simulink model "PlantaMalhaExternaR2018b"  (R2018b)
settings: Solver=VariableStepAuto  StartTime=0.0  StopTime=10.0  RelTol=1e-3
libraries: simulink x1
settings Model: Creator=lucas  LastModifiedBy=vitor
settings DataIOCC: ReturnWorkspaceOutputs=on
settings DebuggingCC: SFMachineParentedDataDiag=error

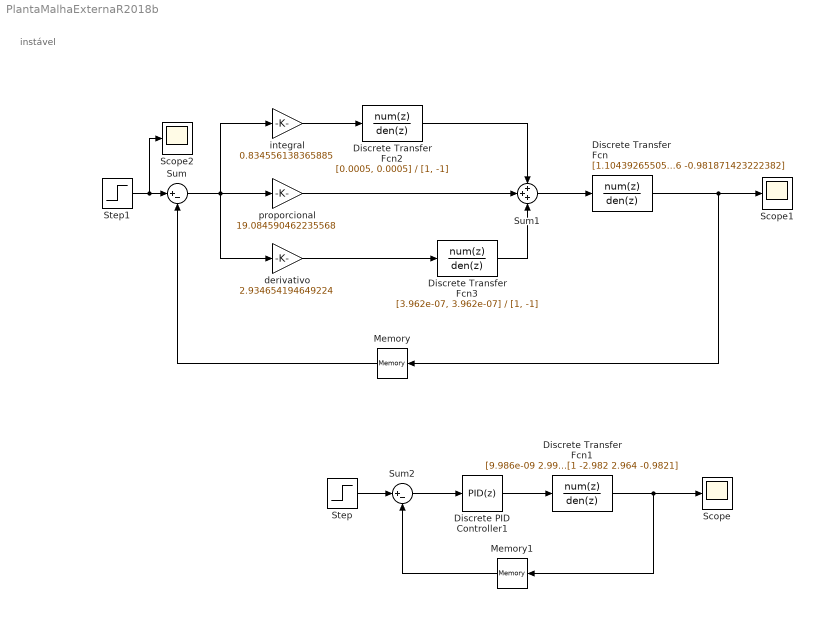
== system PlantaMalhaExternaR2018b ==
  note: instável
  Discrete Transfer Fcn : DiscreteTransferFcn  Numerator=[1.104392655054829e-08 3.313177965164485e-08 3.313177965164485e-08 1.104392655054829e-08]  Denominator=[1 -2.981694681338594 2.963566104560976 -0.981871423222382]  SampleTime=0.001
  Discrete Transfer Fcn1 : DiscreteTransferFcn  Numerator=[9.986e-09 2.996e-08 2.996e-08 9.986e-09]  Denominator=[1 -2.982 2.964 -0.9821]  SampleTime=0.001
  Discrete Transfer Fcn2 : DiscreteTransferFcn  Numerator=[0.0005, 0.0005]  Denominator=[1, -1]
  Discrete Transfer Fcn3 : DiscreteTransferFcn  Numerator=[3.962e-07, 3.962e-07]  Denominator=[1, -1]  SampleTime=0.001
  Discrete PID Controller1 : simulink/Continuous/PID Controller  Controller=PID  Form=Parallel  TimeDomain=Discrete-time  SampleTime=0.001  IntegratorMethod=Forward Euler  FilterMethod=Forward Euler  ControllerParametersSource=internal  P=200  I=0  D=8  UseFilter=on  N=1.824  TunerSelectOption=Transfer Function Based (PID Tuner App)  InitialConditionSource=internal  InitialConditionForIntegrator=0  InitialConditionForFilter=0  DifferentiatorICPrevScaledInput=0  ExternalReset=none  TrackingMode=off  Kt=1  LimitOutput=off  UpperSaturationLimit=inf  LowerSaturationLimit=-inf  LinearizeAsGain=off  AntiWindupMode=none  Kb=1  POutMin=[]  POutMax=[]  IOutMin=[]  IOutMax=[]  DOutMin=[]  DOutMax=[]  NOutMin=[]  NOutMax=[]  SumOutMin=[]  SumOutMax=[]  SaturationOutMin=[]  SaturationOutMax=[]  PParamMin=[]  PParamMax=[]  IParamMin=[]  IParamMax=[]  DParamMin=[]  DParamMax=[]  NParamMin=[]  NParamMax=[]  KbParamMin=[]  KbParamMax=[]  KtParamMin=[]  KtParamMax=[]  KbOutMin=[]  KbOutMax=[]  KtOutMin=[]  KtOutMax=[]  IntegratorOutMin=[]  IntegratorOutMax=[]  FilterOutMin=[]  FilterOutMax=[]  SumI1OutMin=[]  SumI1OutMax=[]  SumI2OutMin=[]  SumI2OutMax=[]  SumI3OutMin=[]  SumI3OutMax=[]  SumI4OutMin=[]  SumI4OutMax=[]  SumDOutMin=[]  SumDOutMax=[]  DifferentiatorOutMin=[]  DifferentiatorOutMax=[]  FilterDiffOutCoefMin=[]  FilterDiffOutCoefMax=[]  ReciprocalOutMin=[]  ReciprocalOutMax=[]  SumDenOutMin=[]  SumDenOutMax=[]  SumNumOutMin=[]  SumNumOutMax=[]  DivideOutMin=[]  DivideOutMax=[]  IntegratorContinuousStateAttributes=''  IntegratorStateMustResolveToSignalObject=off  IntegratorRTWStateStorageClass=Auto  FilterContinuousStateAttributes=''  FilterStateMustResolveToSignalObject=off  FilterRTWStateStorageClass=Auto  ParallelPVariant=InternalParameters  IdealPVariant=Disabled  IVariant=InternalParameters  DVariant=InternalParameters  IntegratorVariant=Discrete  SatVariant=Disabled  AWVariant=Passthrough  PCopyVariant=Disabled  TRVariant=Disabled  FdbkBlocksVariant=Forward  IdealPFdbkVariant=Disabled  SatFdbkVariant=Disabled  DerivativeFilterVariant=ForwardEulerFilter  NVariant=InternalParameters  NCopyVariant=Disabled  FilterICVariant=InternalICsFilter  IntegratorICVariant=InternalICs  ExternalResetVariant=Disabled  TRSumVariant=Passthrough  SumFdbkVariant=Disabled  SumVariant=Sum_PID
  Memory : Memory
  Memory1 : Memory
  Scope : Scope
  Scope1 : Scope
  Scope2 : Scope
  Step : Step  Time=0  After=0.3  SampleTime=0.001
  Step1 : Step  Time=0  After=0.3  SampleTime=0.001
  Sum : Sum  Inputs=|+-
  Sum1 : Sum  Inputs=+++
  Sum2 : Sum  Inputs=|+-
  derivativo : Gain  Gain=2.934654194649224
  integral : Gain  Gain=0.834556138365885
  proporcional : Gain  Gain=19.084590462235568
  wires:
  Discrete Transfer Fcn/1 -> Scope1/1, Memory/1
  Memory/1 -> Sum/2
  Discrete PID Controller1/1 -> Discrete Transfer Fcn1/1
  Memory1/1 -> Sum2/2
  Sum2/1 -> Discrete PID Controller1/1
  Discrete Transfer Fcn1/1 -> Scope/1, Memory1/1
  Step/1 -> Sum2/1
  Step1/1 -> Scope2/1, Sum/1
  Discrete Transfer Fcn3/1 -> Sum1/3
  Sum/1 -> derivativo/1, integral/1, proporcional/1
  proporcional/1 -> Sum1/2
  integral/1 -> Discrete Transfer Fcn2/1
  derivativo/1 -> Discrete Transfer Fcn3/1
  Discrete Transfer Fcn2/1 -> Sum1/1
  Sum1/1 -> Discrete Transfer Fcn/1
